simulink model "Enabled_Triggered_Subsystem"  (R2021a)
settings: Solver=VariableStepAuto  StartTime=0.0  StopTime=10.0  RelTol=1e-3
settings Model: Creator=lenovo  LastModifiedBy=lenovo

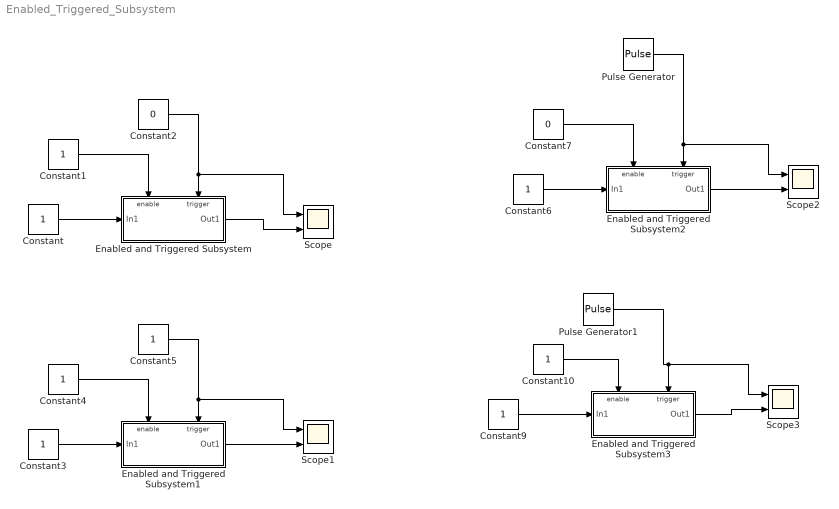
== system Enabled_Triggered_Subsystem ==
  Constant{,1,3..6,9..10} (8 alike) : Constant
  Constant2 : Constant  Value=0
  Constant7 : Constant  Value=0
  Enabled and Triggered Subsystem : Subsystem  TreatAsAtomicUnit=on
  Enabled and Triggered Subsystem1 : Subsystem  TreatAsAtomicUnit=on
  Enabled and Triggered Subsystem2 : Subsystem  TreatAsAtomicUnit=on
  Enabled and Triggered Subsystem3 : Subsystem  TreatAsAtomicUnit=on
  Pulse Generator : DiscretePulseGenerator  PulseType=Time based  PulseWidth=50
  Pulse Generator1 : DiscretePulseGenerator  PulseType=Time based  PulseWidth=50
  Scope{,1..3} (4 alike) : Scope  NumInputPorts=2
  wires:
  Constant/1 -> Enabled and Triggered Subsystem/1(In1)
  Constant2/1 -> Scope/1, Enabled and Triggered Subsystem/Trigger
  Constant1/1 -> Enabled and Triggered Subsystem/Enable
  Constant4/1 -> Enabled and Triggered Subsystem1/Enable
  Constant5/1 -> Scope1/1, Enabled and Triggered Subsystem1/Trigger
  Constant3/1 -> Enabled and Triggered Subsystem1/1(In1)
  Enabled and Triggered Subsystem/1(Out1) -> Scope/2
  Enabled and Triggered Subsystem1/1(Out1) -> Scope1/2
  Enabled and Triggered Subsystem2/1(Out1) -> Scope2/2
  Constant6/1 -> Enabled and Triggered Subsystem2/1(In1)
  Pulse Generator/1 -> Enabled and Triggered Subsystem2/Trigger, Scope2/1
  Constant7/1 -> Enabled and Triggered Subsystem2/Enable
  Constant10/1 -> Enabled and Triggered Subsystem3/Enable
  Pulse Generator1/1 -> Scope3/1, Enabled and Triggered Subsystem3/Trigger
  Constant9/1 -> Enabled and Triggered Subsystem3/1(In1)
  Enabled and Triggered Subsystem3/1(Out1) -> Scope3/2

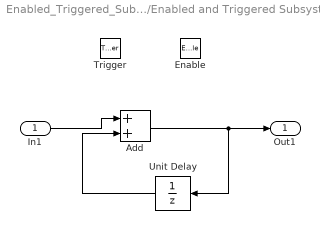
== system Enabled_Triggered_Subsystem/Enabled and Triggered Subsystem ==
  In1 : Inport
  Enable : EnablePort
  Trigger : TriggerPort  VariantControl=(inherit)
  Add : Sum
  Unit Delay : UnitDelay  SampleTime=-1  HasFrameUpgradeWarning=on
  Out1 : Outport
  wires:
  Unit Delay/1 -> Add/2
  Add/1 -> Out1/1, Unit Delay/1
  In1/1 -> Add/1

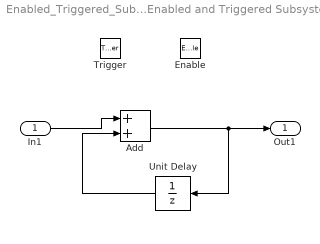
== system Enabled_Triggered_Subsystem/Enabled and Triggered Subsystem1 ==
  In1 : Inport
  Enable : EnablePort
  Trigger : TriggerPort  VariantControl=(inherit)
  Add : Sum
  Unit Delay : UnitDelay  SampleTime=-1  HasFrameUpgradeWarning=on
  Out1 : Outport
  wires:
  In1/1 -> Add/1
  Add/1 -> Unit Delay/1, Out1/1
  Unit Delay/1 -> Add/2

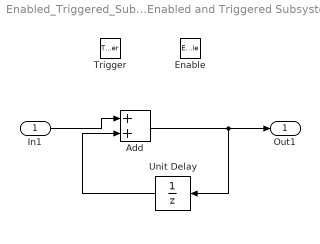
== system Enabled_Triggered_Subsystem/Enabled and Triggered Subsystem2 ==
  In1 : Inport
  Enable : EnablePort
  Trigger : TriggerPort  VariantControl=(inherit)
  Add : Sum
  Unit Delay : UnitDelay  SampleTime=-1  HasFrameUpgradeWarning=on
  Out1 : Outport
  wires:
  Unit Delay/1 -> Add/2
  Add/1 -> Out1/1, Unit Delay/1
  In1/1 -> Add/1

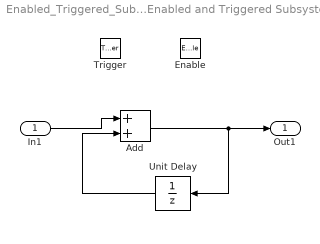
== system Enabled_Triggered_Subsystem/Enabled and Triggered Subsystem3 ==
  In1 : Inport
  Enable : EnablePort
  Trigger : TriggerPort  VariantControl=(inherit)
  Add : Sum
  Unit Delay : UnitDelay  SampleTime=-1  HasFrameUpgradeWarning=on
  Out1 : Outport
  wires:
  In1/1 -> Add/1
  Add/1 -> Unit Delay/1, Out1/1
  Unit Delay/1 -> Add/2
